simulink model "RangeGuidance"  (R2021a)
settings: configuration reference "RPi_ControlRate" (kept outside this file)
settings Model: Creator=barthal  LastModifiedBy=Andy
settings ConfigSetRef: SourceName=RPi_ControlRate  SourceLocation=Base Workspace

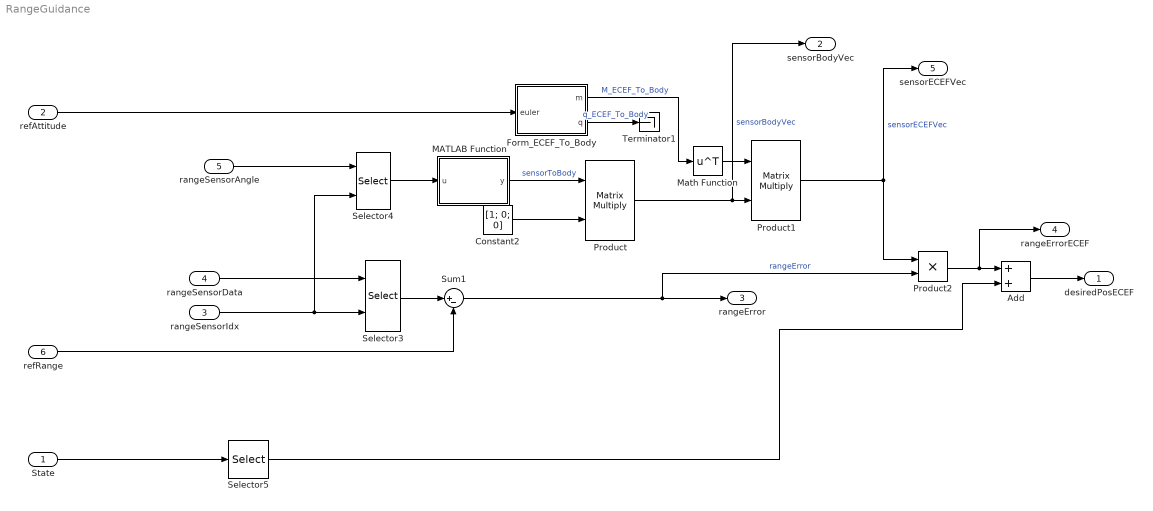
== system RangeGuidance ==
  State : Inport  OutDataTypeStr=double
  refAttitude : Inport  Port=2  OutDataTypeStr=double  PortDimensions=3
  rangeSensorIdx : Inport  Port=3  OutDataTypeStr=double
  rangeSensorData : Inport  Port=4  OutDataTypeStr=double  PortDimensions=4
  rangeSensorAngle : Inport  Port=5  OutDataTypeStr=double  PortDimensions=4
  refRange : Inport  Port=6  OutDataTypeStr=double
  Add : Sum
  Constant2 : Constant  Value=[1; 0; 0]
  Form_ECEF_To_Body : MATLAB Function  TreatAsAtomicUnit=on
  MATLAB Function : MATLAB Function  TreatAsAtomicUnit=on
  Math Function : Math  Operator=transpose  SignedPower=on  SaturateOnIntegerOverflow=on
  Product : Product  Multiplication=Matrix(*)
  Product1 : Product  Multiplication=Matrix(*)
  Product2 : Product
  Selector3 : Selector  InputPortWidth=4  IndexOptions=Index vector (port)  Indices=5  OutputSizes=1
  Selector4 : Selector  InputPortWidth=4  IndexOptions=Index vector (port)  Indices=5  OutputSizes=1
  Selector5 : Selector  InputPortWidth=12  IndexOptions=Index vector (dialog)  Indices=[1:3]  OutputSizes=1
  Sum1 : Sum  Inputs=|+-
  Terminator1 : Terminator
  desiredPosECEF : Outport  VectorParamsAs1DForOutWhenUnconnected=off
  sensorBodyVec : Outport  Port=2  VectorParamsAs1DForOutWhenUnconnected=off
  rangeError : Outport  Port=3  VectorParamsAs1DForOutWhenUnconnected=off
  rangeErrorECEF : Outport  Port=4  VectorParamsAs1DForOutWhenUnconnected=off
  sensorECEFVec : Outport  Port=5  VectorParamsAs1DForOutWhenUnconnected=off
  wires:
  refAttitude/1 -> Form_ECEF_To_Body/1(euler)
  State/1 -> Selector5/1
  rangeSensorIdx/1 -> Selector4/2, Selector3/2
  rangeSensorData/1 -> Selector3/1
  Selector3/1 -> Sum1/1
  Sum1/1 -> Product2/2, rangeError/1  "rangeError"
  rangeSensorAngle/1 -> Selector4/1
  Selector4/1 -> MATLAB Function/1(u)
  MATLAB Function/1(y) -> Product/1  "sensorToBody"
  Constant2/1 -> Product/2
  Product/1 -> sensorBodyVec/1, Product1/2  "sensorBodyVec"
  Product1/1 -> Product2/1, sensorECEFVec/1  "sensorECEFVec"
  Selector5/1 -> Add/2
  Product2/1 -> rangeErrorECEF/1, Add/1
  Add/1 -> desiredPosECEF/1
  Form_ECEF_To_Body/2(q) -> Terminator1/1  "q_ECEF_To_Body"
  Form_ECEF_To_Body/1(m) -> Math Function/1  "M_ECEF_To_Body"
  Math Function/1 -> Product1/1
  refRange/1 -> Sum1/2

== matlab function RangeGuidance/Form_ECEF_To_Body ==
  data: euler input; m output; q output
function [m,q] = fcn(euler)

m = EulerToDCM_321(euler);
q = EulerToquat_321(euler);

== matlab function RangeGuidance/MATLAB Function ==
  data: u input; y output
function y = fcn(u)

y = [cos(u) sin(u) 0; -sin(u) cos(u) 0; 0 0 1];
